simulink library "relay_ANSI_functions_lib"  (Simulink 8.1)
settings: Solver=ode45  StartTime=0.0  StopTime=10.0  RelTol=1e-3
undefined symbols (not defined in the file or in its folder): IOC, TOC, Ts, VRMSLL
settings Model: Creator=RE25624  LastModifiedBy=re25624

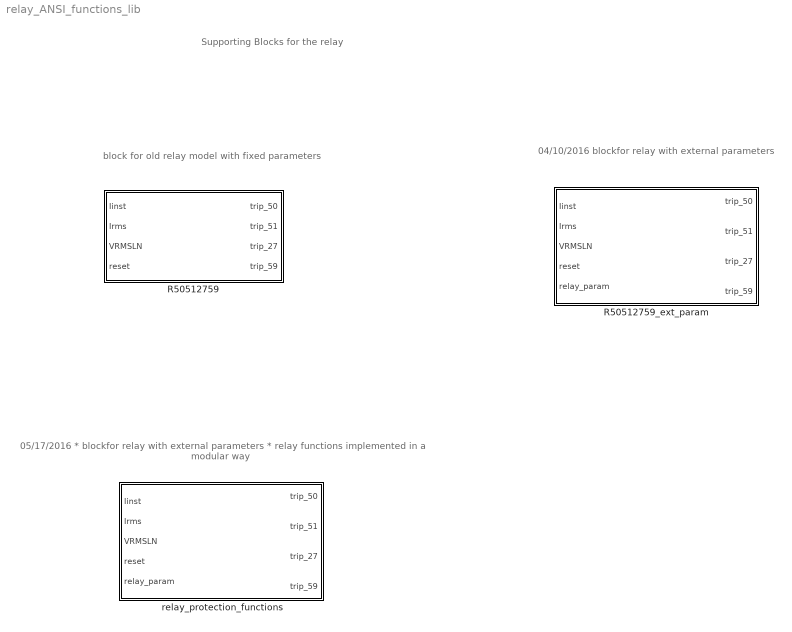
== system relay_ANSI_functions_lib ==
  note: 04/10/2016
      | blockfor relay with external parameters
  note: Supporting Blocks for the relay
  note: block for old relay model with fixed parameters
  note: 05/17/2016
      | * blockfor relay with external parameters
      | * relay functions implemented in a modular way
  R50512759 : Subsystem  mask(Relays 50-51-27-59){VRMSLL=VRMSLL, IOC=IOC, TOC=TOC, Ts=Ts}
      mask prompts: VRMSLL "Nominal Voltage [VRMSLL]"; IOC "IOC Setting [A]"; TOC "TOC Setting [A]"; Ts "Sampling Time [Sec]"
      mask help:
      | This block simulates the behavior of the following relay functions:
      | 1) Instantaneous overcurrent (50)
      | 2) AC inverse time overcurrent (51)
      | 3) Undervoltage (27)
      | 4) Overvoltage (59)
      | It is not suitable for instantaneous earth current relaying.
      | The model neglects the influence CTs since only the logics of the relay are required or the current effort.
  R50512759_ext_param : Subsystem  mask(Relays 50-51-27-59){Ts=Ts}
      mask prompts: Ts "Sampling Time [Sec]"
      mask help:
      | This block simulates the behavior of the following relay functions:
      | 1) Instantaneous overcurrent (50)
      | 2) AC inverse time overcurrent (51)
      | 3) Undervoltage (27)
      | 4) Overvoltage (59)
      | It is not suitable for instantaneous earth current relaying.
      | The model neglects the influence CTs since only the logics of the relay are required or the current effort.
      |
      | The input bus with the relay parameters should be ordered as follows:
      | 1) VRMSLL
      | 2) IOC
      | 3) TOC
      | 4) dV_threshold
      | 5) angle_threshold
      | 6) dF_threshold
  relay_protection_functions : Subsystem  mask(Relays 50-51-27-59){Ts=Ts}
      mask prompts: Ts "Sampling Time [Sec]"
      mask help:
      | This block simulates the behavior of the following relay functions:
      | 1) Instantaneous overcurrent (50)
      | 2) AC inverse time overcurrent (51)
      | 3) Undervoltage (27)
      | 4) Overvoltage (59)
      | It is not suitable for instantaneous earth current relaying.
      | The model neglects the influence CTs since only the logics of the relay are required or the current effort.
      |
      | The input bus with the relay parameters should be ordered as follows:
      | 1) VRMSLL
      | 2) IOC
      | 3) TOC
      | 4) dV_threshold
      | 5) angle_threshold
      | 6) dF_threshold

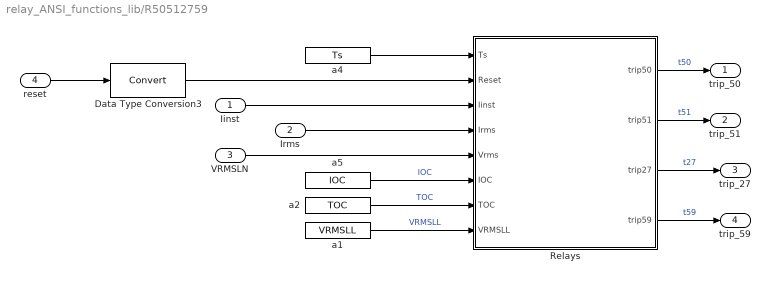
== system relay_ANSI_functions_lib/R50512759 ==
  Iinst : Inport
  Irms : Inport  Port=2
  VRMSLN : Inport  Port=3
  reset : Inport  Port=4
  Data Type Conversion3 : DataTypeConversion
  Relays : MATLAB Function  TreatAsAtomicUnit=on
  a1 : Constant  Value=VRMSLL
  a2 : Constant  Value=TOC
  a4 : Constant  Value=Ts
  a5 : Constant  Value=IOC
  trip_50 : Outport
  trip_51 : Outport  Port=2
  trip_27 : Outport  Port=3
  trip_59 : Outport  Port=4
  wires:
  Data Type Conversion3/1 -> Relays/2(Reset)
  Relays/2(trip51) -> trip_51/1  "t51"
  Relays/1(trip50) -> trip_50/1  "t50"
  Relays/4(trip59) -> trip_59/1  "t59"
  Relays/3(trip27) -> trip_27/1  "t27"
  a4/1 -> Relays/1(Ts)
  a1/1 -> Relays/8(VRMSLL)  "VRMSLL"
  VRMSLN/1 -> Relays/5(Vrms)
  Irms/1 -> Relays/4(Irms)
  a2/1 -> Relays/7(TOC)  "TOC"
  Iinst/1 -> Relays/3(Iinst)
  a5/1 -> Relays/6(IOC)  "IOC"
  reset/1 -> Data Type Conversion3/1

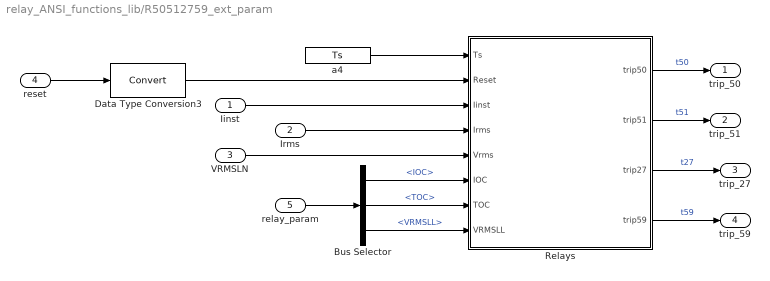
== system relay_ANSI_functions_lib/R50512759_ext_param ==
  Iinst : Inport
  Irms : Inport  Port=2
  VRMSLN : Inport  Port=3
  reset : Inport  Port=4
  relay_param : Inport  Port=5
  Bus Selector : BusSelector  OutputSignals=IOC,TOC,VRMSLL
  Data Type Conversion3 : DataTypeConversion
  Relays : MATLAB Function  TreatAsAtomicUnit=on
  a4 : Constant  Value=Ts
  trip_50 : Outport
  trip_51 : Outport  Port=2
  trip_27 : Outport  Port=3
  trip_59 : Outport  Port=4
  wires:
  relay_param/1 -> Bus Selector/1
  Data Type Conversion3/1 -> Relays/2(Reset)
  Relays/2(trip51) -> trip_51/1  "t51"
  Relays/1(trip50) -> trip_50/1  "t50"
  Relays/4(trip59) -> trip_59/1  "t59"
  Relays/3(trip27) -> trip_27/1  "t27"
  a4/1 -> Relays/1(Ts)
  Bus Selector/3 -> Relays/8(VRMSLL)  "<VRMSLL>"
  VRMSLN/1 -> Relays/5(Vrms)
  Irms/1 -> Relays/4(Irms)
  Bus Selector/2 -> Relays/7(TOC)  "<TOC>"
  Iinst/1 -> Relays/3(Iinst)
  Bus Selector/1 -> Relays/6(IOC)  "<IOC>"
  reset/1 -> Data Type Conversion3/1

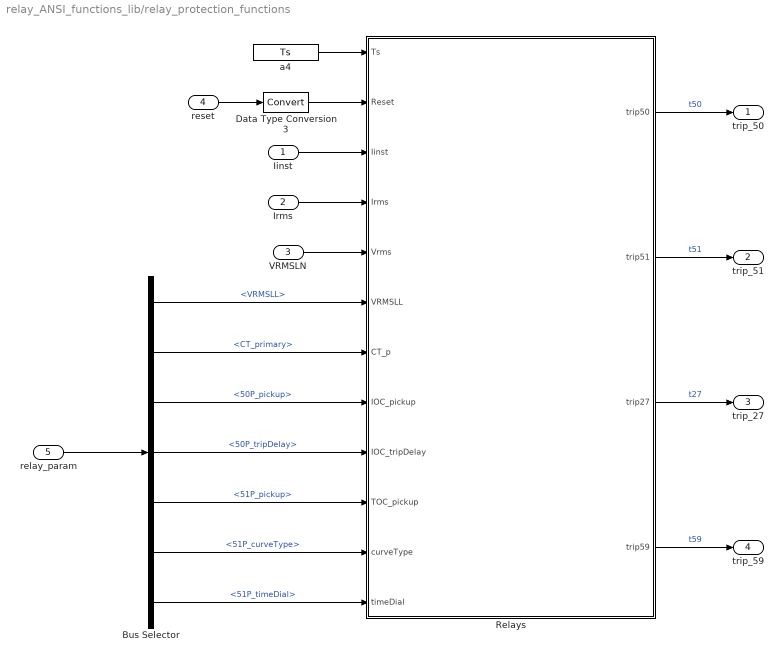
== system relay_ANSI_functions_lib/relay_protection_functions ==
  Iinst : Inport
  Irms : Inport  Port=2
  VRMSLN : Inport  Port=3
  reset : Inport  Port=4
  relay_param : Inport  Port=5
  Bus Selector : BusSelector  OutputSignals=VRMSLL,CT_primary,50P_pickup,50P_tripDelay,51P_pickup,51P_curveType,51P_timeDial
  Data Type Conversion3 : DataTypeConversion
  Relays : MATLAB Function  TreatAsAtomicUnit=on
  a4 : Constant  Value=Ts
  trip_50 : Outport
  trip_51 : Outport  Port=2
  trip_27 : Outport  Port=3
  trip_59 : Outport  Port=4
  wires:
  Iinst/1 -> Relays/3(Iinst)
  Irms/1 -> Relays/4(Irms)
  Bus Selector/7 -> Relays/12(timeDial)  "<51P_timeDial>"
  Bus Selector/6 -> Relays/11(curveType)  "<51P_curveType>"
  Bus Selector/5 -> Relays/10(TOC_pickup)  "<51P_pickup>"
  Bus Selector/4 -> Relays/9(IOC_tripDelay)  "<50P_tripDelay>"
  Bus Selector/3 -> Relays/8(IOC_pickup)  "<50P_pickup>"
  Bus Selector/2 -> Relays/7(CT_p)  "<CT_primary>"
  Bus Selector/1 -> Relays/6(VRMSLL)  "<VRMSLL>"
  reset/1 -> Data Type Conversion3/1
  VRMSLN/1 -> Relays/5(Vrms)
  a4/1 -> Relays/1(Ts)
  Relays/3(trip27) -> trip_27/1  "t27"
  Relays/4(trip59) -> trip_59/1  "t59"
  Relays/1(trip50) -> trip_50/1  "t50"
  Relays/2(trip51) -> trip_51/1  "t51"
  Data Type Conversion3/1 -> Relays/2(Reset)
  relay_param/1 -> Bus Selector/1

== matlab function relay_protection_functions/Relays ==
  data: Ts input double; trip50 output double; Reset input double; Iinst input double; Irms input double; Vrms input double; VRMSLL input double; CT_p input double; trip51 output double; trip27 output double; IOC_pickup input double; trip59 output double; IOC_tripDelay input double; TOC_pickup input double; curveType input double; timeDial input double
% CREATED BY: REYNALDO SALCEDO
% LAST CHANGE BY : REYNALDO SALCEDO
% GROUP: 73
% DATE MODIFIED  : 05/17/2016
%

function [trip50, trip51, trip27, trip59] = relay_elements(Ts, Reset, Iinst, Irms, Vrms, VRMSLL,...
    CT_p, IOC_pickup, IOC_tripDelay, TOC_pickup, curveType, timeDial)
%#codegen

% initialize or reset the trip signals
persistent R50 R51 R27 R59
if isempty(R51) || Reset
    R50=false;
    R51=false;
    R59=false;
    R27=false;
end

% applying turns CT ratio - assuming protection CT
Iinst = Iinst * (5/CT_p);
Irms = Irms * (5/CT_p);

% latch for true signals
if ~(R50==true || R51==true)
    % calling external function expressing relay protection elements
    T50 = relay_ANSI_50P_script(Ts, Iinst , IOC_pickup, IOC_tripDelay);
    T51 = relay_ANSI_51P_script(Ts, Irms, TOC_pickup, curveType, timeDial);
    [r] = relay_ANSI_2759_script(Ts, Vrms, VRMSLL);
    
    R50 = T50;
    R51 = T51;
    R27 = r.trip27;
    R59 = r.trip59;
end

trip50 = R50; % latched
trip51 = R51; % latched
trip27 = R27; % not latched
trip59 = R59; % not latched

== matlab function R50512759/Relays ==
  data: Ts input double; trip50 output double; Reset input double; Iinst input double; Irms input double; Vrms input double; IOC input double; trip51 output double; trip27 output double; TOC input double; VRMSLL input double; trip59 output double
% CREATED BY: REYNALDO SALCEDO
% LAST CHANGE BY : REYNALDO SALCEDO
% GROUP: 73
% DATE MODIFIED  : 04/13/2016
%

function [trip50, trip51, trip27, trip59] = relays_50512759(Ts, Reset, Iinst, Irms, Vrms, IOC, TOC, VRMSLL)
%#codegen

% initialize or reset the trip signals
persistent R50 R51 R27 R59
if isempty(R51) || Reset
    R50=false;
    R51=false;
    R59=false;
    R27=false;
end

% latch for true signals
if ~(R50==true || R51==true)
    % calling external function
    r = relay_ANSI_50512759_script(Ts, Iinst, Irms, Vrms, IOC, TOC, VRMSLL);
    R50 = r.trip50;
    R51 = r.trip51;
    R27 = r.trip27;
    R59 = r.trip59;
end

trip50 = R50; % latched
trip51 = R51; % latched
trip27 = R27; % not latched
trip59 = R59; % not latched

== matlab function R50512759_ext_param/Relays ==
  data: Ts input double; trip50 output double; Reset input double; Iinst input double; Irms input double; Vrms input double; IOC input double; trip51 output double; trip27 output double; TOC input double; VRMSLL input double; trip59 output double
% CREATED BY: REYNALDO SALCEDO
% LAST CHANGE BY : REYNALDO SALCEDO
% GROUP: 73
% DATE MODIFIED  : 04/13/2016
%

function [trip50, trip51, trip27, trip59] = relays_50512759(Ts, Reset, Iinst, Irms, Vrms, IOC, TOC, VRMSLL)
%#codegen

% initialize or reset the trip signals
persistent R50 R51 R27 R59
if isempty(R51) || Reset
    R50=false;
    R51=false;
    R59=false;
    R27=false;
end

% latch for true signals
if ~(R50==true || R51==true)
    % calling external function
    r = relay_ANSI_50512759_script(Ts, Iinst, Irms, Vrms, IOC, TOC, VRMSLL);
    R50 = r.trip50;
    R51 = r.trip51;
    R27 = r.trip27;
    R59 = r.trip59;
end

trip50 = R50; % latched
trip51 = R51; % latched
trip27 = R27; % not latched
trip59 = R59; % not latched
